simulink model "test7"  (R2018a)
settings: Solver=VariableStepAuto  StartTime=0.0  StopTime=10.0  RelTol=1e-3
settings Model: Creator=thomas  LastModifiedBy=thomas

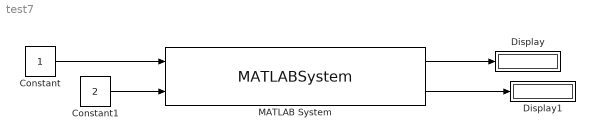
== system test7 ==
  Constant : Constant  OutDataTypeStr=uint8
  Constant1 : Constant  Value=2  OutDataTypeStr=uint8
  Display : Display
  Display1 : Display
  MATLAB System : MATLABSystem  System=sim7  ts=1e-3  SimulateUsing=Code generation  plcIP=0.0.0.0  plcRack=0  plcSlot=1  writeDB=[ 1001, 1002 ]  writePos=[ 0, 0 ]  writeSize=[ 1, 1 ]  readDB=[ 1001, 1002 ]  readPos=[ 0, 0 ]  readSize=[ 1, 1 ]
      mask Type: sim7
      mask Display:
      | disp(['snap7 PLC' char(10) 'IP: 0.0.0.0' char(10) 'Rack: 0 Slot:1' char(10) 'Ts: 1ms']);
      | port_label('input',1,'1001[0:0]');
      | port_label('input',2,'1002[0:0]');
      | port_label('output',1,'1001[0:0]');
      | port_label('output',2,'1002[0:0]');
  wires:
  Constant/1 -> MATLAB System/1
  Constant1/1 -> MATLAB System/2
  MATLAB System/1 -> Display/1
  MATLAB System/2 -> Display1/1
